simulink model "KP_Collect_UCS"  (R2025b)
settings: Solver=VariableStepAuto  StartTime=0.0  StopTime=tspan  FixedStep=dt_sim  RelTol=1e-3
model workspace (MAT data in the model file):
  socvcb = containers.Map
  socvcb.serialization.keys = {}
  socvcb.serialization.values = {}
  socvcb.serialization.uniformity = 0
  socvcb.serialization.keyType = 'double'
  socvcb.serialization.valueType = 'any'
undefined symbols (not defined in the file): background_pose, distort_coefL, doExactPerspective, dt_sample, dt_sim, exactDistance_KP, exactPhi_KP, exactTheta_KP, gate1_Pose, gate_center, k_L, keyPointsWorld, M_UCSToWorld, M_WorldToUCS, numKeypoints, numPerspectives, perspectives, rel_CamPose_L, rel_CamPose_L_UCS, rel_CamPose_R_UCS, Sim3dSensor, startDelay_KP
libraries: sim3dlib x12, sim3dcameralib x2
settings Model: Creator=Liam  LastModifiedBy=Liam

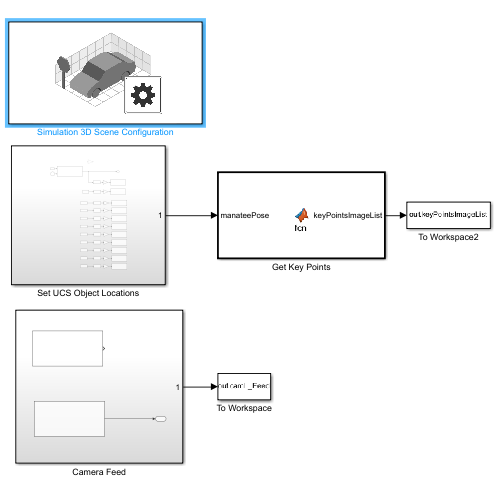
[thumbnail: Simulink's stored preview of the top-level diagram]
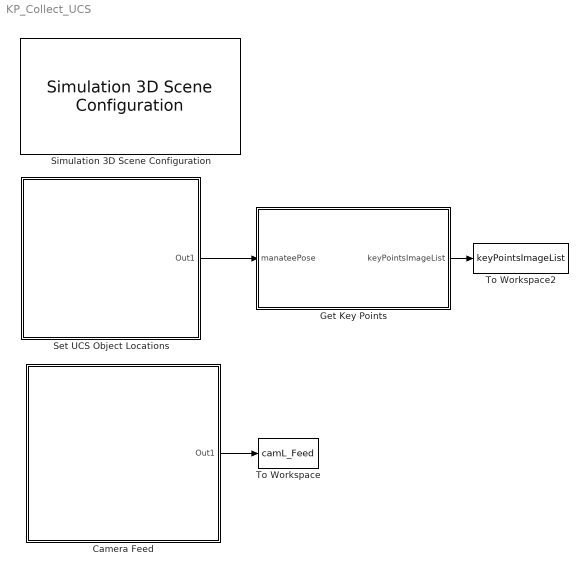
== system KP_Collect_UCS ==
  Camera Feed : Subsystem  Priority=1
  Get Key Points : MATLAB Function  TreatAsAtomicUnit=on
  Set UCS Object Locations : Subsystem  Priority=1
  Simulation 3D Scene Configuration : sim3dlib/Simulation 3D Scene Configuration  Priority=0  ProjectFormat=Unreal Executable  SceneDesc=Straight road  ProjectName=C:\Users\Liam\OneDrive\Documents\GitHub\SimulinkPlant\DROP UCS PACKAGED BUILD HERE\EllingtonPoolSim.exe  ScenePath=/Game/Prop_Test_Level  UEProjPath=C:\Users\Liam\OneDrive\Documents\GitHub\Vision_Sim\Unreal\UnrealProjects\SimulinkCoSimulation\EllingtonPoolSim\EllingtonPoolSim.uproject  EnableOpenDRIVE=off  vehTagList={'Custom';'Scene Origin'}  vehTag=Scene Origin  AttachedCameraRelativeTranslation=[0 0 0]  FreeCameraDefaultInitialTranslation=[-6, 0, 2]  AttachedCameraRelativeRotation=[0 0 0]  FreeCameraDefaultInitialRotation=[0, -15, 0]  ViewpointName=Custom  FreeCameraInitialTranslation=[0, 0, 0]  ViewpointTranslation=[0 0 0]  FreeCameraInitialRotation=[0, 0, 0]  ViewpointRotation=[0 0 0]  OpVisEn=off  Ts=dt_sample  EnableWindow=on  EnableRemoteAccess=off  EnableWeather=off  SunAzimuth=90  SunAltitude=40.0  EnableGeospatialSun=off  Latitude=0  Longitude=0  Date=2023-01-01  Time=10:30:00  GeoTimeZone=-5.0  SunDaylightSaving=off  wind=1  clouds=10  EnableVolumetricClouds=off  CloudCoverage=0  CloudAltitude=6  fog=0  rain=0  RaindropsEffect=off  SnowDensity=0  EnableGeospatial=off  TilesetSource=Earth terrain  UseTrueOrigin=off  OriginHeight=200  OriginLatitude=40.744652  OriginLongitude=-73.988864  MapStyle=Aerial  AdditionalAssetIDs=[]  UseAdvancedSunSky=off  SolarTime=11  TimeZone=-5  Day=21  Month=9  Year=2022  UseDaylightSavingTime=on  DSTStartDay=10  DSTStartMonth=3  DSTEndDay=3  DSTEndMonth=11  DSTSwitchHour=2  sensorTag=MainCamera1  sensorId=1  sensorName=MainCamera1  mountLoc=Origin  offsetFlag=off  tmountOffset=[0, 0, 0]  rmountOffset=[0, 0, 0]  HorizontalResolution=1280  VerticalResolution=720  HorizontalFOV=60  mountPoint=[0 0 0]  mountOrientation=[0 0 0]  aMode=3  ID=1  GeoTrigger=Inactive  ViewNameList={'Custom'}  ViewTranslationList={'[0 0 0]'}  ViewRotationList={'[0 0 0]'}
      settings: LibrarySourceBlock=drivingsim3d/Simulation 3D Scene Configuration
  To Workspace : ToWorkspace  VariableName=camL_Feed  SampleTime=dt_sample*2
      settings: Save2DSignal=2-D array (concatenate along first dimension)
  To Workspace2 : ToWorkspace  VariableName=keyPointsImageList  SampleTime=dt_sample*2
      settings: Save2DSignal=2-D array (concatenate along first dimension)
  wires:
  Get Key Points/1(keyPointsImageList) -> To Workspace2/1
  Set UCS Object Locations/1(Out1) -> Get Key Points/1(manateePose)
  Camera Feed/1(Out1) -> To Workspace/1

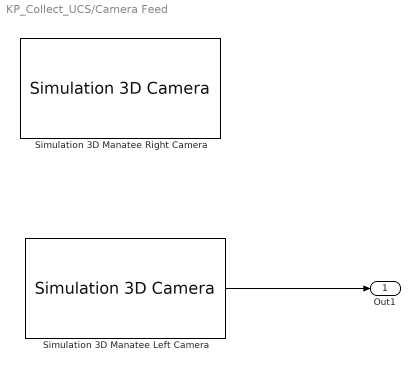
== system KP_Collect_UCS/Camera Feed ==
  Simulation 3D Manatee Left Camera : sim3dcameralib/Simulation 3D Camera  Priority=1  sensorTag=Sim3dSensor�  sensorId=1  sensorName=Sim3dSensor�  vehTagList={'Scene Origin'}  vehTag=Scene Origin  CoordinateSystem=Default  mountLoc=Origin  offsetFlag=on  tmountOffset=rel_CamPose_L_UCS(1:3) / 100  extTmount=off  rmountOffset=rel_CamPose_L_UCS(4:6)  extRmount=off  FocalLength=[2.97 / 0.0028, 2.97 / 0.0028]  OpticalCenter=[960, 540]  ImageSize=[1080, 1920]  RadialDistortion=[0.33 0.16]  TangentialDistortion=[0 0]  SensorSkew=0  VisualizeFieldOfView=off  FieldOfViewRange=61  DepthOutportEnabled=off  SemanticOutportEnabled=off  TransformOutportEnabled=off  SampleTime=dt_sample  mountPoint=[0.4 -0.125 0.15]  mountOrientation=[0 0 0]  aMode=5  ID=1
      settings: LibrarySourceBlock=sl3dlib/Simulation 3D/Sensors/Simulation 3D Camera
  Simulation 3D Manatee Right Camera : sim3dcameralib/Simulation 3D Camera  Priority=1  sensorTag=Sim3dSensor�  sensorId=2  sensorName=Sim3dSensor�  vehTagList={'Scene Origin'}  vehTag=Scene Origin  CoordinateSystem=Default  mountLoc=Origin  offsetFlag=on  tmountOffset=rel_CamPose_R_UCS(1:3) / 100  extTmount=off  rmountOffset=rel_CamPose_R_UCS(4:6)  extRmount=off  FocalLength=[2.97 / 0.0028, 2.97 / 0.0028]  OpticalCenter=[960, 540]  ImageSize=[1080, 1920]  RadialDistortion=[0.33 0.16]  TangentialDistortion=[0 0]  SensorSkew=0  VisualizeFieldOfView=off  FieldOfViewRange=61  DepthOutportEnabled=off  SemanticOutportEnabled=off  TransformOutportEnabled=off  SampleTime=dt_sample  mountPoint=[0.4 0.125 0.15]  mountOrientation=[0 0 0]  aMode=5  ID=2
      settings: LibrarySourceBlock=sl3dlib/Simulation 3D/Sensors/Simulation 3D Camera
  Out1 : Outport
  wires:
  Simulation 3D Manatee Left Camera/1 -> Out1/1

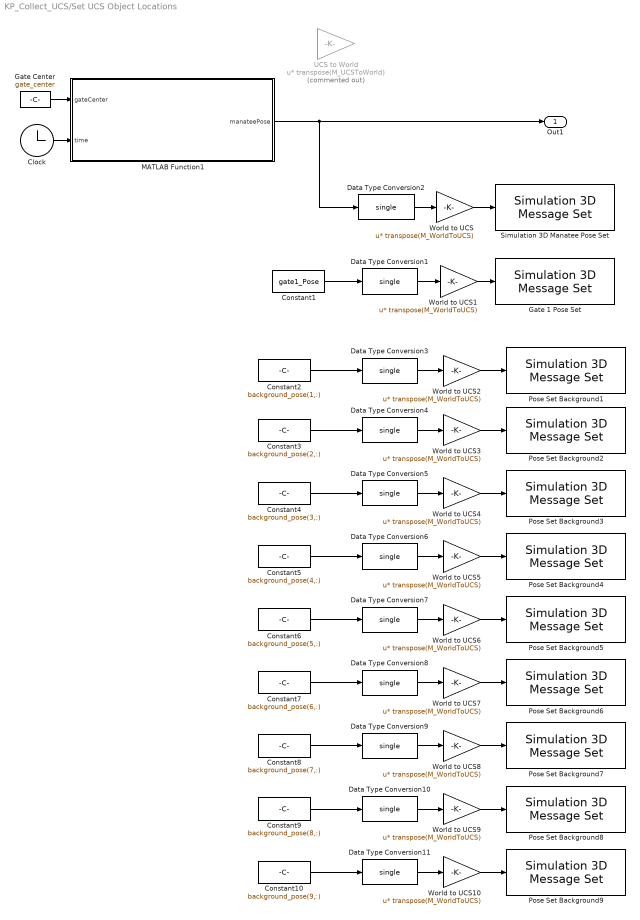
== system KP_Collect_UCS/Set UCS Object Locations ==
  Clock : Clock
  Constant1 : Constant  Value=gate1_Pose  VectorParams1D=off  OutDataTypeStr=single
  Constant10 : Constant  Value=background_pose(9,:)  VectorParams1D=off  OutDataTypeStr=single
  Constant2 : Constant  Value=background_pose(1,:)  VectorParams1D=off  OutDataTypeStr=single
  Constant3 : Constant  Value=background_pose(2,:)  VectorParams1D=off  OutDataTypeStr=single
  Constant4 : Constant  Value=background_pose(3,:)  VectorParams1D=off  OutDataTypeStr=single
  Constant5 : Constant  Value=background_pose(4,:)  VectorParams1D=off  OutDataTypeStr=single
  Constant6 : Constant  Value=background_pose(5,:)  VectorParams1D=off  OutDataTypeStr=single
  Constant7 : Constant  Value=background_pose(6,:)  VectorParams1D=off  OutDataTypeStr=single
  Constant8 : Constant  Value=background_pose(7,:)  VectorParams1D=off  OutDataTypeStr=single
  Constant9 : Constant  Value=background_pose(8,:)  VectorParams1D=off  OutDataTypeStr=single
  Data Type Conversion{1..11} (11 alike) : DataTypeConversion  OutDataTypeStr=single  SaturateOnIntegerOverflow=off  RndMeth=Floor
  Gate 1 Pose Set : sim3dlib/Simulation 3D Message Set  Priority=-1  SigName=Gate1PoseSet  Ts=dt_sample  aMode=0
      settings: LibrarySourceBlock=aerolibsim3d/Simulation 3D Message Set
  Gate Center : Constant  Value=gate_center  VectorParams1D=off  OutDataTypeStr=single  SampleTime=-1
  MATLAB Function1 : MATLAB Function  TreatAsAtomicUnit=on
  Pose Set Background1 : sim3dlib/Simulation 3D Message Set  Priority=-1  SigName=Background1PoseSet  Ts=dt_sample  aMode=0
      settings: LibrarySourceBlock=aerolibsim3d/Simulation 3D Message Set
  Pose Set Background2 : sim3dlib/Simulation 3D Message Set  Priority=-1  SigName=Background2PoseSet  Ts=dt_sample  aMode=0
      settings: LibrarySourceBlock=aerolibsim3d/Simulation 3D Message Set
  Pose Set Background3 : sim3dlib/Simulation 3D Message Set  Priority=-1  SigName=Background3PoseSet  Ts=dt_sample  aMode=0
      settings: LibrarySourceBlock=aerolibsim3d/Simulation 3D Message Set
  Pose Set Background4 : sim3dlib/Simulation 3D Message Set  Priority=-1  SigName=Background4PoseSet  Ts=dt_sample  aMode=0
      settings: LibrarySourceBlock=aerolibsim3d/Simulation 3D Message Set
  Pose Set Background5 : sim3dlib/Simulation 3D Message Set  Priority=-1  SigName=Background5PoseSet  Ts=dt_sample  aMode=0
      settings: LibrarySourceBlock=aerolibsim3d/Simulation 3D Message Set
  Pose Set Background6 : sim3dlib/Simulation 3D Message Set  Priority=-1  SigName=Background6PoseSet  Ts=dt_sample  aMode=0
      settings: LibrarySourceBlock=aerolibsim3d/Simulation 3D Message Set
  Pose Set Background7 : sim3dlib/Simulation 3D Message Set  Priority=-1  SigName=Background7PoseSet  Ts=dt_sample  aMode=0
      settings: LibrarySourceBlock=aerolibsim3d/Simulation 3D Message Set
  Pose Set Background8 : sim3dlib/Simulation 3D Message Set  Priority=-1  SigName=Background8PoseSet  Ts=dt_sample  aMode=0
      settings: LibrarySourceBlock=aerolibsim3d/Simulation 3D Message Set
  Pose Set Background9 : sim3dlib/Simulation 3D Message Set  Priority=-1  SigName=Background9PoseSet  Ts=dt_sample  aMode=0
      settings: LibrarySourceBlock=aerolibsim3d/Simulation 3D Message Set
  Simulation 3D Manatee Pose Set : sim3dlib/Simulation 3D Message Set  Priority=-1  SigName=ManateePoseSet  Ts=dt_sample  aMode=0
      settings: LibrarySourceBlock=aerolibsim3d/Simulation 3D Message Set
  UCS to World : Gain  Commented=on  Gain=transpose(M_UCSToWorld)  Multiplication=Matrix(u*K)
  World to UCS{,1..10} (11 alike) : Gain  Gain=transpose(M_WorldToUCS)  Multiplication=Matrix(u*K)
  Out1 : Outport
  wires:
  Gate Center/1 -> MATLAB Function1/1(gateCenter)
  Clock/1 -> MATLAB Function1/2(time)
  Constant1/1 -> Data Type Conversion1/1
  World to UCS1/1 -> Gate 1 Pose Set/1
  Data Type Conversion1/1 -> World to UCS1/1
  Data Type Conversion2/1 -> World to UCS/1
  World to UCS/1 -> Simulation 3D Manatee Pose Set/1
  MATLAB Function1/1(manateePose) -> Data Type Conversion2/1, Out1/1
  Data Type Conversion3/1 -> World to UCS2/1
  World to UCS2/1 -> Pose Set Background1/1
  Constant2/1 -> Data Type Conversion3/1
  Constant3/1 -> Data Type Conversion4/1
  Data Type Conversion4/1 -> World to UCS3/1
  World to UCS3/1 -> Pose Set Background2/1
  Constant4/1 -> Data Type Conversion5/1
  Data Type Conversion5/1 -> World to UCS4/1
  World to UCS4/1 -> Pose Set Background3/1
  Constant5/1 -> Data Type Conversion6/1
  Data Type Conversion6/1 -> World to UCS5/1
  World to UCS5/1 -> Pose Set Background4/1
  Constant6/1 -> Data Type Conversion7/1
  Data Type Conversion7/1 -> World to UCS6/1
  World to UCS6/1 -> Pose Set Background5/1
  Constant7/1 -> Data Type Conversion8/1
  Data Type Conversion8/1 -> World to UCS7/1
  World to UCS7/1 -> Pose Set Background6/1
  Constant8/1 -> Data Type Conversion9/1
  Data Type Conversion9/1 -> World to UCS8/1
  World to UCS8/1 -> Pose Set Background7/1
  Constant9/1 -> Data Type Conversion10/1
  Data Type Conversion10/1 -> World to UCS9/1
  World to UCS9/1 -> Pose Set Background8/1
  Constant10/1 -> Data Type Conversion11/1
  Data Type Conversion11/1 -> World to UCS10/1
  World to UCS10/1 -> Pose Set Background9/1

== matlab function KP_Collect_UCS/Set UCS Object Locations/MATLAB Function1 ==
  settings: updateMethod=DISCRETE  sampleTime=dt_sample
  data: gateCenter input; manateePose output; exactDistance_KP parameter; exactPhi_KP parameter; exactTheta_KP parameter; doExactPerspective parameter; perspectives parameter; numPerspectives parameter; time input; dt_sample parameter; dt_sim parameter; startDelay_KP parameter
function manateePose = manateeViewPointGate(gateCenter, exactDistance_KP, exactPhi_KP, exactTheta_KP, doExactPerspective, perspectives, numPerspectives, time, dt_sample, dt_sim, startDelay_KP)
if (doExactPerspective == true)
    x = exactDistance_KP * sin(exactTheta_KP) * cos(exactPhi_KP);
    y = exactDistance_KP * sin(exactTheta_KP) * sin(exactPhi_KP);
    z = exactDistance_KP * cos(exactTheta_KP);
    manateeRoll = 0;
    manateePitch = (pi / 2 - exactTheta_KP);
    manateeYaw = exactPhi_KP - pi;
    
    manateePose = [(gateCenter(1) + x) (gateCenter(2) + y) (gateCenter(3) + z) manateeRoll manateePitch  manateeYaw];
else
    iterator = int32(time * 1000 / dt_sample * dt_sim);
    manateePose = single(zeros(1,6));
    i = (iterator - startDelay_KP + 1) / 2;
    if (i > 0 && i <= numPerspectives && mod(i,1) == 0)
        x = perspectives(i, 1);
        y = perspectives(i, 2);
        z = perspectives(i, 3);
        manateeRoll = perspectives(i, 4);
        manateePitch = perspectives(i, 5);
        manateeYaw = perspectives(i, 6);
        manateePose = [(x) (y) (z) manateeRoll manateePitch  manateeYaw];
    end
end

== matlab function KP_Collect_UCS/Get Key Points ==
  settings: updateMethod=DISCRETE  sampleTime=dt_sample
  data: manateePose input; rel_CamPose_L parameter; keyPointsWorld parameter; k_L parameter; distort_coefL parameter; numKeypoints parameter; keyPointsImageList output
function keyPointsImageList = fcn(manateePose,rel_CamPose_L, keyPointsWorld, k_L, distort_coefL, numKeypoints)

keyPointsImageList = zeros(1,13);
keyPointsImageList(1) = 0;

for i = 1:numKeypoints
    keyPoint = worldToImageCoord(keyPointsWorld(i,:), manateePose, rel_CamPose_L, k_L, distort_coefL);
    q = i*3 - 1;
    keyPointsImageList(q) = keyPoint(1);
    keyPointsImageList(q+1) = keyPoint(2);
    keyPointsImageList(q+2) = keyPoint(3);
end
